simulink model "Vienna"  (R2024b)
settings: Solver=ode23t  StartTime=0.0  StopTime=2  RelTol=1e-3
undefined symbols (not defined in the file): acdc, Cur_loop_upper_limit_acdc, DiscIntNeverNeededParam, kp_ff, kr_ff, Tsim, vdc_fbk_filter
libraries: simulink x9, spsDiodeLib x6, spsMosfetLib x6, spsSeriesRLCBranchLib x5, spsVoltageMeasurementLib x4, spsMeanLib x4, spsCurrentMeasurementLib x3, spsControlledVoltageSourceLib x3, spsRMSLib x2, spsThreePhaseSourceLib x1, spsTHDLib x1, spsTriangleGeneratorLib x1
(part 1 of 2)
settings Model: Creator=PAGHDMD  LastModifiedBy=PAGHDMD
settings OptimizationCC: ReuseModelBlockBuffer=off
settings RTWCC: GPUComputeCapability=3.5

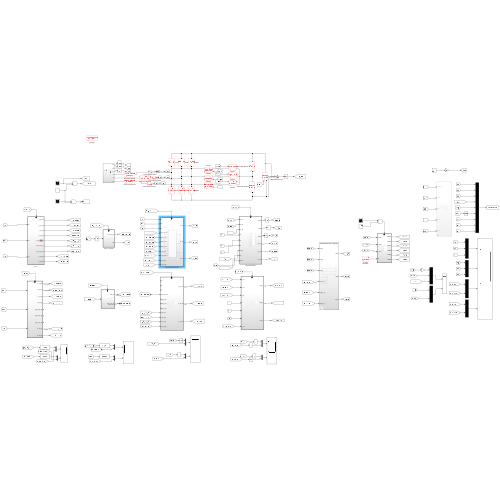
[thumbnail: Simulink's stored preview of the top-level diagram]
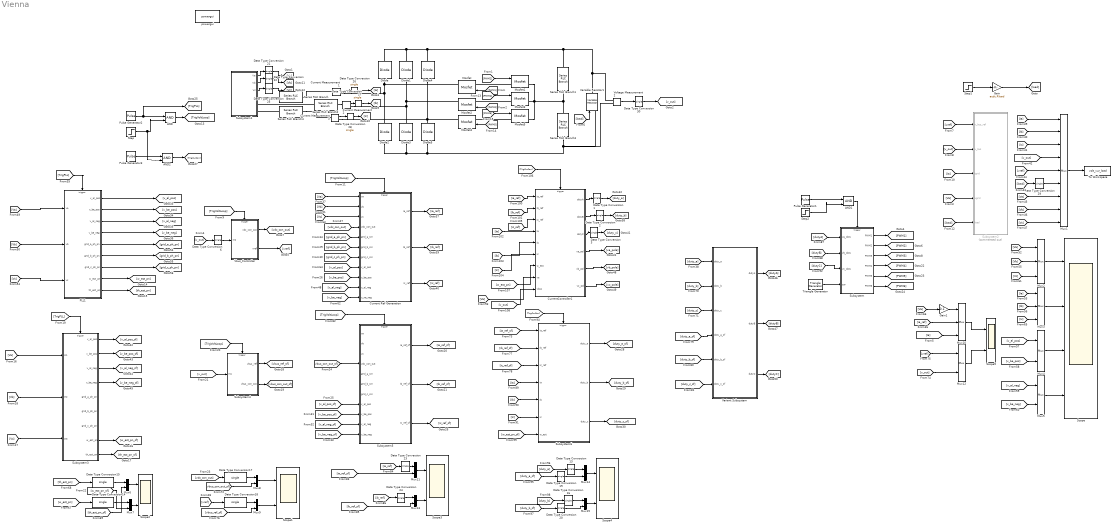
== system Vienna ==
  AND : Logic  IconShape=distinctive  AllPortsSameDT=off  OutDataTypeStr=boolean
  AND1 : Logic  IconShape=distinctive  AllPortsSameDT=off  OutDataTypeStr=boolean
  AND2 : Logic  IconShape=distinctive  AllPortsSameDT=off  OutDataTypeStr=boolean
  Current Measurement1 : spsCurrentMeasurementLib/Current Measurement  PhasorSimulation=off  OutputType=Complex  PSBequivalent=0
  Current Measurement2 : spsCurrentMeasurementLib/Current Measurement  PhasorSimulation=off  OutputType=Complex  PSBequivalent=0
  Current Measurement3 : spsCurrentMeasurementLib/Current Measurement  PhasorSimulation=off  OutputType=Complex  PSBequivalent=0
  Current Ref Generation : Subsystem
  CurrentController1 : Subsystem
  Data Type Conversion{1..3,6,13..30} (22 alike) : DataTypeConversion  OutDataTypeStr=single  SaturateOnIntegerOverflow=off  RndMeth=Floor
  Diode{,1..5} (6 alike) : spsDiodeLib/Diode  Ron=0.001  Lon=0  Vf=0.8  IC=0  UseSnubber=0  Rs=500  Cs=250e-9  Measurements=off
  Gain : Gain  Gain=acdc.Rload
  Gain1 : Gain  Gain=0.1
  Mosfet{,1..5} (6 alike) : spsMosfetLib/Mosfet  Ron=50e-3  Lon=0  Rd=0.01  Vfd=0  IC=0  Rs=1e5  Cs=inf  Measurements=on
  Mux1 : Mux  Inputs=9
  Mux10 : Mux  Inputs=3
  Mux{4..9,11..15} (11 alike) : Mux  Inputs=2
  Mux2 : Mux  Inputs=3
  Mux3 : Mux  Inputs=3
  PLL1 : Subsystem
  Pulse Generator1 : DiscretePulseGenerator  PulseType=Time based  Period=Tsim  PulseWidth=5
  Pulse Generator2 : DiscretePulseGenerator  PulseType=Time based  Period=acdc.Tvolt_loop  PulseWidth=5
  Pulse Generator3 : DiscretePulseGenerator  PulseType=Time based  Period=acdc.Tcur_loop  PulseWidth=5
  Scope : Scope  NumInputPorts=4
  Scope{1..5} (5 alike) : Scope  NumInputPorts=2
  Series RLC Branch : spsSeriesRLCBranchLib/Series RLC Branch  LConnTagsString=__new0  RConnTagsString=__new0  BranchType=RL  Resistance=acdc.L_ESR  Inductance=acdc.L  SetiL0=off  InitialCurrent=0  Capacitance=1e-6  Setx0=off  InitialVoltage=0  Measurements=None
  Series RLC Branch1 : spsSeriesRLCBranchLib/Series RLC Branch  LConnTagsString=__new0  RConnTagsString=__new0  BranchType=C  Resistance=1  Inductance=40e-6  SetiL0=off  InitialCurrent=0  Capacitance=acdc.C/2  Setx0=on  InitialVoltage=acdc.Vac_ll_rms*sqrt(2)/2  Measurements=None
  Series RLC Branch2 : spsSeriesRLCBranchLib/Series RLC Branch  LConnTagsString=__new0  RConnTagsString=__new0  BranchType=RL  Resistance=acdc.L_ESR  Inductance=acdc.L  SetiL0=off  InitialCurrent=0  Capacitance=1e-6  Setx0=off  InitialVoltage=0  Measurements=None
  Series RLC Branch3 : spsSeriesRLCBranchLib/Series RLC Branch  LConnTagsString=__new0  RConnTagsString=__new0  BranchType=C  Resistance=1  Inductance=40e-6  SetiL0=off  InitialCurrent=0  Capacitance=acdc.C/2  Setx0=on  InitialVoltage=acdc.Vac_ll_rms*sqrt(2)/2  Measurements=None
  Series RLC Branch4 : spsSeriesRLCBranchLib/Series RLC Branch  LConnTagsString=__new0  RConnTagsString=__new0  BranchType=RL  Resistance=acdc.L_ESR  Inductance=acdc.L  SetiL0=off  InitialCurrent=0  Capacitance=1e-6  Setx0=off  InitialVoltage=0  Measurements=None
  Step : Step  Time=0.02  SampleTime=0
  Step1 : Step  Time=0.5  Before=1  After=2  SampleTime=0
  Step2 : Step  Time=0.02  SampleTime=0
  Subsystem : Subsystem
  Subsystem1 : Subsystem
  Subsystem2 : Subsystem  Commented=on
  Subsystem3 : Subsystem
  Subsystem4 : Subsystem
  Subsystem5 : Subsystem
  Subsystem6 : Subsystem
  To Workspace : ToWorkspace  VariableName=volt_vur_load  SaveFormat=Timeseries  SampleTime=-1
      settings: Decimation=100
  Triangle Generator : spsTriangleGeneratorLib/Triangle Generator  Freq=acdc.Fs  Phase=0  Ts=Tsim
  Variable Resistor1 : spsVariableResistorLib/Variable Resistor  Rabsmin=1e-3
      settings: LibrarySourceBlock=sps_lib/Passives/Variable Resistor
  Variant Subsystem : Subsystem  Variant=on
  Vbus_Controller : Subsystem
  Voltage Measurement2 : spsVoltageMeasurementLib/Voltage Measurement  PhasorSimulation=off  OutputType=Complex  PSBequivalent=0
  powergui : spspowerguiLib/powergui  Priority=1  SimulationMode=Discrete  SampleTime=Tsim  frequency=60  Iterations=50  frequencyindice=0  Pbase=100e6  ErrMax=1e-4  UnitsV=kV  UnitsW=MW  buscounter=0  FunctionMessages=off  echomessages=off  EnableUseOfTLC=off  CurrentSourceSwitches=off  DisableSnubberDevices=off  DisableRonSwitches=off  DisableVfSwitches=off  DisplayEquations=off  AutomaticDiscreteSolvers=off  SolverType=Tustin/Backward Euler (TBE)  Interpol=off  ExternalGateDelay=off  methode=off  Ts=100  x0status=blocks  SPID=on  SwTol=0  HookPort=off  NonlinearTolerance=1e-4  nMaxIteration=100  ContinueOnMaxIteration=off  RestoreLinks=warning  ResistiveCurrentMeasurement=off  Frange=[0:2:500]  Ylog=off  Xlog=on  ShowGrid=off  save=off  variable=ZData  structure=0  ZoomFFT=off  StartTime=0.0  cycles=1  DisplayStyle=1  fundamental=60  FreqAxis=off  MaxFrequency=1000  frequencyindicesteady=1  RmsSteady=1  display=off
  wires:
  Voltage Measurement2/1 -> Data Type Conversion30/1
  Current Measurement1/1 -> Data Type Conversion26/1
  [PWM1] -> Mosfet/1
  [PWM2] -> Mosfet1/1
  Subsystem/1(PWM1) -> [PWM1]
  Subsystem/2(PWM2) -> [PWM2]
  Step1/1 -> Gain/1
  Gain/1 -> [load]
  [load] -> Variable Resistor1/1
  [vref] -> Subsystem2/1(v_bus_ref)
  [v_out] -> Subsystem2/2(v_bus)
  [Ia] -> Subsystem2/3(igrid)
  [Va] -> Subsystem2/4(vgrid)
  [load] -> Subsystem2/5(load)
  [v_out] -> Data Type Conversion6/1
  Vbus_Controller/2(vref) -> [vref]
  Subsystem1/1(Va) -> Data Type Conversion21/1
  [PWM3] -> Mosfet2/1
  [PWM4] -> Mosfet3/1
  [PWM5] -> Mosfet4/1
  [PWM6] -> Mosfet5/1
  Current Measurement2/1 -> Data Type Conversion27/1
  Current Measurement3/1 -> Data Type Conversion28/1
  Subsystem1/2(Vb) -> Data Type Conversion22/1
  Subsystem1/3(Vc) -> Data Type Conversion25/1
  Pulse Generator2/1 -> [TrigPLL], AND/1
  AND/1 -> [TrigVoltLoop]
  [TrigVoltLoop] -> Vbus_Controller/Trigger
  Subsystem/3(PWM3) -> [PWM3]
  Subsystem/4(PWM4) -> [PWM4]
  Subsystem/5(PWM5) -> [PWM5]
  Subsystem/6(PWM6) -> [PWM6]
  Pulse Generator1/1 -> AND1/1
  Triangle Generator/1 -> Subsystem/4(car)
  [Ia] -> Mux1/1
  [Ib] -> Mux1/2
  [Ic] -> Mux1/3
  [v_out] -> Mux1/4
  [load] -> Data Type Conversion29/1
  Mux1/1 -> To Workspace/1
  [vref] -> Mux1/5
  [Va] -> Mux1/7
  [Vb] -> Mux1/8
  [Vc] -> Mux1/9
  [TrigPLL] -> PLL1/Trigger
  Mux2/1 -> Scope/1
  [Va] -> Mux2/1
  [Vb] -> Mux2/2
  [v_al_pos] -> Mux4/1
  [v_be_pos] -> Mux4/2
  [v_al_neg] -> Mux5/1
  [v_be_neg] -> Mux5/2
  Mux3/1 -> Scope/2
  Mux4/1 -> Scope/3
  Mux5/1 -> Scope/4
  [Vc] -> Mux2/3
  [dutyA] -> Subsystem/1(va_duty)
  [dutyB] -> Subsystem/2(vb_duty)
  [dutyC] -> Subsystem/3(vc_duty)
  Mux10/1 -> Scope5/1
  [ia_ref] -> Mux10/2
  [Va] -> Gain1/1
  Gain1/1 -> Mux10/1
  Vbus_Controller/1(vdc_con_out) -> [vdc_con_out]
  [Ia] -> Mux10/3
  [TrigVoltLoop] -> Current Ref Generation/Trigger
  Current Ref Generation/1(ia_ref) -> [ia_ref]
  Current Ref Generation/2(ib_ref) -> [ib_ref]
  Current Ref Generation/3(ic_ref) -> [ic_ref]
  [vdc_con_out] -> Current Ref Generation/4(vdc_con_out)
  [grid_a_ph_pn] -> Current Ref Generation/5(grid_a_sin)
  [grid_b_ph_pn] -> Current Ref Generation/6(grid_b_sin)
  [grid_c_ph_pn] -> Current Ref Generation/7(grid_c_sin)
  Mux12/1 -> Scope5/2
  [v_out] -> Mux12/2
  [vref] -> Mux12/1
  Step2/1 -> AND1/2
  AND1/1 -> Subsystem/Trigger
  [v_al_pos] -> Current Ref Generation/8(v_al_pos)
  [v_be_pos] -> Current Ref Generation/9(v_be_pos)
  [v_al_neg] -> Current Ref Generation/10(v_al_neg)
  [v_be_neg] -> Current Ref Generation/11(v_ne_neg)
  [Ia] -> Mux3/1
  [Ib] -> Mux3/2
  [Ic] -> Mux3/3
  [Va] -> PLL1/1(va)
  [Vb] -> PLL1/2(vb)
  [Vc] -> PLL1/3(vc)
  PLL1/1(v_al_pos) -> [v_al_pos]
  PLL1/2(v_be_pos) -> [v_be_pos]
  PLL1/3(v_al_neg) -> [v_al_neg]
  PLL1/5(grid_a_ph_pn) -> [grid_a_ph_pn]
  PLL1/4(v_be_neg) -> [v_be_neg]
  PLL1/6(grid_b_ph_pn) -> [grid_b_ph_pn]
  PLL1/7(grid_c_ph_pn) -> [grid_c_ph_pn]
  [Va] -> Subsystem3/1(In1)
  [Vb] -> Subsystem3/2(In2)
  [Vc] -> Subsystem3/3(In3)
  [TrigPLL] -> Subsystem3/Trigger
  PLL1/8(w_est_pn) -> [w_est_pn]
  PLL1/9(th_est_pn) -> [th_est_pn]
  Mux7/1 -> Scope2/2
  Mux6/1 -> Scope2/1
  Data Type Conversion14/1 -> Mux7/1
  Data Type Conversion15/1 -> Mux6/1
  [TrigVoltLoop] -> Subsystem4/Trigger
  [vdc_con_out] -> Data Type Conversion17/1
  Mux8/1 -> Scope1/1
  [v_out] -> Subsystem4/1(In1)
  Data Type Conversion17/1 -> Mux8/1
  Mux9/1 -> Scope1/2
  [vref] -> Data Type Conversion18/1
  Data Type Conversion18/1 -> Mux9/1
  [w_est_pn] -> Data Type Conversion14/1
  [th_est_pn] -> Data Type Conversion15/1
  Subsystem3/8(w_est_pn) -> [w_est_pn_sf]
  Subsystem3/9(th_est_pn) -> [th_est_pn_sf]
  [w_est_pn_sf] -> Mux7/2
  [th_est_pn_sf] -> Mux6/2
  Subsystem4/2(vbus_con_out) -> [vbus_con_out_sf]
  Subsystem4/1(vbus_ref) -> [vbus_ref_sf]
  [vbus_con_out_sf] -> Mux8/2
  [vbus_ref_sf] -> Mux9/2
  Subsystem5/1(ia_ref_sf) -> [ia_ref_sf]
  Subsystem5/2(ib_ref_sf) -> [ib_ref_sf]
  Subsystem5/3(ic_ref_sf) -> [ic_ref_sf]
  [TrigVoltLoop] -> Subsystem5/Trigger
  [v_al_pos_sf] -> Subsystem5/8(v_al_pos)
  [v_be_pos_sf] -> Subsystem5/9(v_be_pos)
  [v_al_neg_sf] -> Subsystem5/10(v_al_neg)
  [v_be_neg_sf] -> Subsystem5/11(v_be_neg)
  Mux11/1 -> Scope3/1
  Mux13/1 -> Scope3/2
  [ia_ref] -> Data Type Conversion23/1
  [ia_ref_sf] -> Mux11/2
  [ib_ref_sf] -> Mux13/2
  [vbus_con_out_sf] -> Subsystem5/4(vdc_con_out)
  Data Type Conversion23/1 -> Mux11/1
  [ib_ref] -> Data Type Conversion24/1
  Data Type Conversion24/1 -> Mux13/1
  [ib_ref_sf] -> Subsystem6/2(ib_ref)
  [ic_ref_sf] -> Subsystem6/3(ic_ref)
  [ia_ref_sf] -> Subsystem6/1(ia_ref)
  [Ia] -> Subsystem6/4(ia)
  [Ib] -> Subsystem6/5(ib)
  [Ic] -> Subsystem6/6(ic)
  Pulse Generator3/1 -> AND2/1
  Step/1 -> AND2/2, AND/2
  AND2/1 -> [TrigCurCon]
  [TrigCurCon] -> Subsystem6/Trigger
  Subsystem6/1(duty_a) -> [duty_a_sf]
  Subsystem6/2(duty_b) -> [duty_b_sf]
  Subsystem6/3(duty_c) -> [duty_c_sf]
  [duty_a_sf] -> Data Type Conversion19/1
  [duty_b_sf] -> Data Type Conversion20/1
  Mux15/1 -> Scope4/2
  Mux14/1 -> Scope4/1
  [duty_b] -> Data Type Conversion16/1
  [duty_a] -> Data Type Conversion13/1
  [w_est_pn_sf] -> Subsystem6/7(w_est)
  CurrentController1/4(va_pol) -> [va_pole]
  CurrentController1/3(dutyC) -> Data Type Conversion3/1
  [w_est_pn] -> CurrentController1/7(w_est)
  CurrentController1/6(vc_pol) -> [vc_pole]
  CurrentController1/1(dutyA) -> Data Type Conversion1/1
  [ib_ref] -> CurrentController1/2(ib_ref)
  [ic_ref] -> CurrentController1/3(ic_ref)
  CurrentController1/5(vb_pol) -> [vb_pole]
  [ia_ref] -> CurrentController1/1(ia_ref)
  CurrentController1/2(dutyB) -> Data Type Conversion2/1
  [TrigCurCon] -> CurrentController1/Trigger
  Subsystem3/1(v_al_pos) -> [v_al_pos_sf]
  Subsystem3/2(v_be_pos) -> [v_be_pos_sf]
  Subsystem3/3(v_al_neg) -> [v_al_neg_sf]
  Subsystem3/4(v_be_neg) -> [v_be_neg_sf]
  Data Type Conversion13/1 -> Mux14/1
  Data Type Conversion16/1 -> Mux15/1
  Data Type Conversion19/1 -> Mux14/2
  Data Type Conversion20/1 -> Mux15/2
  [Va] -> Current Ref Generation/1(va)
  [Vb] -> Current Ref Generation/2(vb)
  [Vc] -> Current Ref Generation/3(vc)
  Data Type Conversion6/1 -> Vbus_Controller/1(In2)
  [Ia] -> CurrentController1/4(ia)
  [Ib] -> CurrentController1/5(ib)
  [Ic] -> CurrentController1/6(ic)
  Data Type Conversion21/1 -> [Va]
  Data Type Conversion22/1 -> [Vb]
  Data Type Conversion25/1 -> [Vc]
  Data Type Conversion26/1 -> [Ia]
  Data Type Conversion27/1 -> [Ib]
  Data Type Conversion28/1 -> [Ic]
  Data Type Conversion29/1 -> Mux1/6
  Data Type Conversion30/1 -> [v_out]
  Data Type Conversion1/1 -> [duty_a]
  Data Type Conversion2/1 -> [duty_b]
  Data Type Conversion3/1 -> [duty_c]
  [duty_c_sf] -> Variant Subsystem/6(duty_c_sf)
  [duty_a] -> Variant Subsystem/1(duty_a)
  [duty_b] -> Variant Subsystem/2(duty_b)
  [duty_c] -> Variant Subsystem/3(duty_c)
  [duty_b_sf] -> Variant Subsystem/5(duty_b_sf)
  [duty_a_sf] -> Variant Subsystem/4(duty_a_sf)
  Variant Subsystem/1(dutyA) -> [dutyA]
  Variant Subsystem/2(dutyB) -> [dutyB]
  Variant Subsystem/3(dutyC) -> [dutyC]
  [Va] -> CurrentController1/8(va)
  [v_out] -> CurrentController1/9(vbus)
  connections:
  Diode2/RConn1 -- Current Measurement1/RConn1 -- Mosfet/RConn1 -- Diode/LConn1
  Diode2/LConn1 -- Diode3/LConn1 -- Diode5/LConn1 -- Series RLC Branch3/RConn1 -- Voltage Measurement2/LConn2 -- Variable Resistor1/LConn1
  Voltage Measurement2/LConn1 -- Diode4/RConn1 -- Diode1/RConn1 -- Diode/RConn1 -- Series RLC Branch1/LConn1 -- Variable Resistor1/RConn1
  Mosfet1/RConn1 -- Series RLC Branch3/LConn1 -- Series RLC Branch1/RConn1 -- Mosfet5/RConn1 -- Mosfet3/RConn1
  Current Measurement1/LConn1 -- Series RLC Branch/RConn1
  Mosfet1/LConn1 -- Mosfet/LConn1
  Subsystem1/RConn1 -- Series RLC Branch/LConn1
  Series RLC Branch2/LConn1 -- Subsystem1/RConn2
  Series RLC Branch4/LConn1 -- Subsystem1/RConn3
  Diode1/LConn1 -- Diode3/RConn1 -- Current Measurement2/RConn1 -- Mosfet2/RConn1
  Diode4/LConn1 -- Mosfet4/RConn1 -- Current Measurement3/RConn1 -- Diode5/RConn1
  Mosfet3/LConn1 -- Mosfet2/LConn1
  Mosfet5/LConn1 -- Mosfet4/LConn1
  Series RLC Branch2/RConn1 -- Current Measurement2/LConn1
  Series RLC Branch4/RConn1 -- Current Measurement3/LConn1

== system Vienna/Current Ref Generation ==
  va : Inport
  vb : Inport  Port=2
  vc : Inport  Port=3
  vdc_con_out : Inport  Port=4
  grid_a_sin : Inport  Port=5
  grid_b_sin : Inport  Port=6
  grid_c_sin : Inport  Port=7
  v_al_pos : Inport  Port=8
  v_be_pos : Inport  Port=9
  v_al_neg : Inport  Port=10
  v_ne_neg : Inport  Port=11
  Trigger : TriggerPort  VariantControl=(inherit)  PortDimensions=1
  Variant Subsystem : Subsystem  Variant=on
  ia_ref : Outport  OutDataTypeStr=single
  ib_ref : Outport  Port=2  OutDataTypeStr=single
  ic_ref : Outport  Port=3  OutDataTypeStr=single
  wires:
  Variant Subsystem/2(ib_ref) -> ib_ref/1
  va/1 -> Variant Subsystem/1(va)
  vb/1 -> Variant Subsystem/2(vb)
  vc/1 -> Variant Subsystem/3(vc)
  vdc_con_out/1 -> Variant Subsystem/4(vdc_con_out)
  grid_a_sin/1 -> Variant Subsystem/5(grid_a_sin)
  grid_b_sin/1 -> Variant Subsystem/6(grid_b_sin)
  grid_c_sin/1 -> Variant Subsystem/7(grid_c_sin)
  Variant Subsystem/1(ia_ref) -> ia_ref/1
  Variant Subsystem/3(ic_ref) -> ic_ref/1
  v_al_pos/1 -> Variant Subsystem/8(v_al_pos)
  v_be_pos/1 -> Variant Subsystem/9(v_be_pos)
  v_al_neg/1 -> Variant Subsystem/10(v_al_neg)
  v_ne_neg/1 -> Variant Subsystem/11(v_be_neg)

== system Vienna/CurrentController1 ==
  ia_ref : Inport
  ib_ref : Inport  Port=2
  ic_ref : Inport  Port=3
  ia : Inport  Port=4
  ib : Inport  Port=5
  ic : Inport  Port=6
  w_est : Inport  Port=7
  va : Inport  Port=8
  vbus : Inport  Port=9
  Trigger : TriggerPort  VariantControl=(inherit)  PortDimensions=1
  Variant Subsystem : Subsystem  Variant=on
  dutyA : Outport
  dutyB : Outport  Port=2
  dutyC : Outport  Port=3
  va_pol : Outport  Port=4
  vb_pol : Outport  Port=5
  vc_pol : Outport  Port=6
  wires:
  ia_ref/1 -> Variant Subsystem/1(ia_ref)
  ib_ref/1 -> Variant Subsystem/2(ib_ref)
  ic_ref/1 -> Variant Subsystem/3(ic_ref)
  ib/1 -> Variant Subsystem/5(ib)
  w_est/1 -> Variant Subsystem/7(w_est)
  ia/1 -> Variant Subsystem/4(ia)
  ic/1 -> Variant Subsystem/6(ic)
  Variant Subsystem/1(dutyA) -> dutyA/1
  Variant Subsystem/2(dutyB) -> dutyB/1
  Variant Subsystem/3(dutyC) -> dutyC/1
  Variant Subsystem/4(va_pol) -> va_pol/1
  Variant Subsystem/5(vb_pol) -> vb_pol/1
  Variant Subsystem/6(vc_pol) -> vc_pol/1
  va/1 -> Variant Subsystem/8(va)
  vbus/1 -> Variant Subsystem/9(vbus)

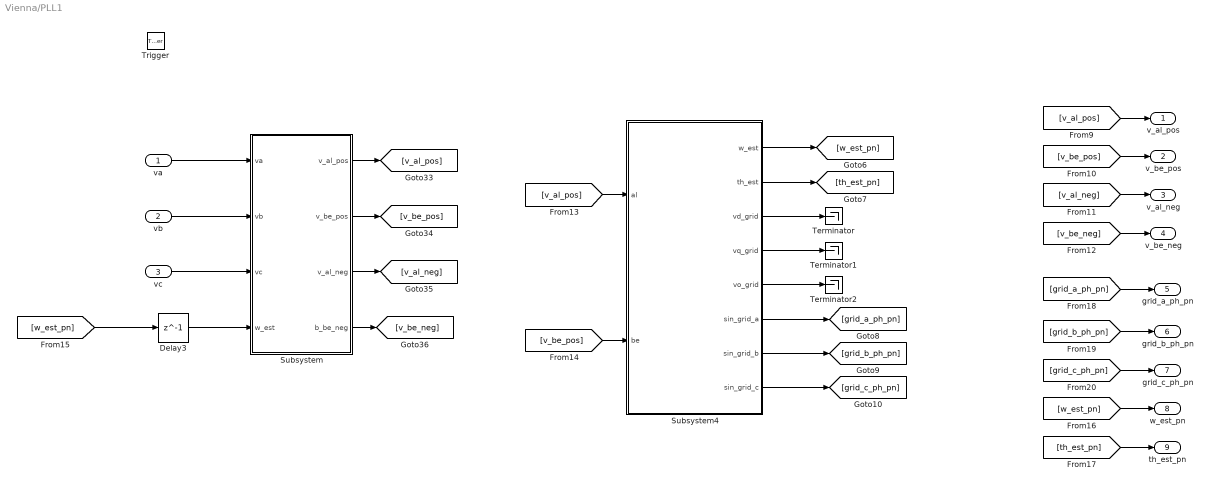
== system Vienna/PLL1 ==
  va : Inport
  vb : Inport  Port=2
  vc : Inport  Port=3
  Trigger : TriggerPort  VariantControl=(inherit)  PortDimensions=1
  Delay3 : Delay  DelayLength=1
  Subsystem : Subsystem
  Subsystem4 : Subsystem
  Terminator : Terminator
  Terminator1 : Terminator
  Terminator2 : Terminator
  v_al_pos : Outport
  v_be_pos : Outport  Port=2
  v_al_neg : Outport  Port=3
  v_be_neg : Outport  Port=4
  grid_a_ph_pn : Outport  Port=5
  grid_b_ph_pn : Outport  Port=6
  grid_c_ph_pn : Outport  Port=7
  w_est_pn : Outport  Port=8
  th_est_pn : Outport  Port=9
  wires:
  [w_est_pn] -> Delay3/1
  va/1 -> Subsystem/1(va)
  vb/1 -> Subsystem/2(vb)
  vc/1 -> Subsystem/3(vc)
  Subsystem/1(v_al_pos) -> [v_al_pos]
  Subsystem/2(v_be_pos) -> [v_be_pos]
  Subsystem/3(v_al_neg) -> [v_al_neg]
  Subsystem/4(b_be_neg) -> [v_be_neg]
  Delay3/1 -> Subsystem/4(w_est)
  [v_al_pos] -> v_al_pos/1
  [v_be_pos] -> v_be_pos/1
  [v_al_neg] -> v_al_neg/1
  [v_be_neg] -> v_be_neg/1
  [v_al_pos] -> Subsystem4/1(al)
  [v_be_pos] -> Subsystem4/2(be)
  Subsystem4/1(w_est) -> [w_est_pn]
  Subsystem4/6(sin_grid_a) -> [grid_a_ph_pn]
  Subsystem4/7(sin_grid_b) -> [grid_b_ph_pn]
  Subsystem4/8(sin_grid_c) -> [grid_c_ph_pn]
  Subsystem4/2(th_est) -> [th_est_pn]
  [w_est_pn] -> w_est_pn/1
  [th_est_pn] -> th_est_pn/1
  [grid_a_ph_pn] -> grid_a_ph_pn/1
  [grid_b_ph_pn] -> grid_b_ph_pn/1
  [grid_c_ph_pn] -> grid_c_ph_pn/1
  Subsystem4/3(vd_grid) -> Terminator/1
  Subsystem4/4(vq_grid) -> Terminator1/1
  Subsystem4/5(vo_grid) -> Terminator2/1

== system Vienna/Subsystem ==
  va_duty : Inport
  vb_duty : Inport  Port=2
  vc_duty : Inport  Port=3
  car : Inport  Port=4
  Trigger : TriggerPort  VariantControl=(inherit)  PortDimensions=1
  Variant Subsystem : Subsystem  Variant=on
  PWM1 : Outport
  PWM2 : Outport  Port=2
  PWM3 : Outport  Port=3
  PWM4 : Outport  Port=4
  PWM5 : Outport  Port=5
  PWM6 : Outport  Port=6
  wires:
  va_duty/1 -> Variant Subsystem/1(va_duty)
  vb_duty/1 -> Variant Subsystem/2(vb_duty)
  vc_duty/1 -> Variant Subsystem/3(vc_duty)
  car/1 -> Variant Subsystem/4(car)
  Variant Subsystem/1(PWM1) -> PWM1/1
  Variant Subsystem/2(PWM2) -> PWM2/1
  Variant Subsystem/3(PWM3) -> PWM3/1
  Variant Subsystem/4(PWM4) -> PWM4/1
  Variant Subsystem/5(PWM5) -> PWM5/1
  Variant Subsystem/6(PWM6) -> PWM6/1

== system Vienna/Subsystem1 ==
  Scope : Scope  NumInputPorts=3
  Subsystem : Subsystem
  Subsystem1 : Subsystem
  Three-Phase Source : spsThreePhaseSourceLib/Three-Phase Source  InternalConnection=Yn  VoltagePhases=on  Voltage=acdc.Vac_ll_rms  PhaseAngle=0  Voltage_phases="[acdc.va  acdc.vb acdc.vc]"  PhaseAngles_phases="[acdc.va_ph  acdc.vb_ph  acdc.vc_ph]"  Frequency=acdc.Fac  NonIdealSource=off  SpecifyImpedance=off  Resistance=0.8929  Inductance=16.58e-3  ShortCircuitLevel=100e6  BaseVoltage=25e3  XRratio=7  BusType=swing  Pref=10e3  Qref=0  Prefabc=[10e3, 10e3, 10e3]  Qrefabc=[0, 0, 0]  Qmin=-inf  Qmax=inf
  Voltage Measurement1 : spsVoltageMeasurementLib/Voltage Measurement  PhasorSimulation=off  OutputType=Complex  PSBequivalent=0
  Voltage Measurement2 : spsVoltageMeasurementLib/Voltage Measurement  PhasorSimulation=off  OutputType=Complex  PSBequivalent=0
  Voltage Measurement3 : spsVoltageMeasurementLib/Voltage Measurement  PhasorSimulation=off  OutputType=Complex  PSBequivalent=0
  A : PMIOPort  Side=Right
  B : PMIOPort  Port=2  Side=Right
  C : PMIOPort  Port=3  Side=Right
  Va : Outport
  Vb : Outport  Port=2
  Vc : Outport  Port=3
  wires:
  Voltage Measurement1/1 -> Va/1
  Voltage Measurement2/1 -> Vb/1
  Voltage Measurement3/1 -> Vc/1
  Subsystem1/1(s) -> Subsystem/1(s), Scope/1
  Subsystem1/2(s1) -> Subsystem/2(s1), Scope/2
  Subsystem1/3(s2) -> Subsystem/3(s2), Scope/3
  connections:
  A/RConn1 -- Subsystem/RConn1 -- Voltage Measurement1/LConn1
  Voltage Measurement3/LConn1 -- C/RConn1 -- Subsystem/RConn3
  Voltage Measurement2/LConn1 -- Subsystem/RConn2 -- B/RConn1
  Voltage Measurement1/LConn2 -- Voltage Measurement3/LConn2 -- Subsystem/RConn4 -- Voltage Measurement2/LConn2

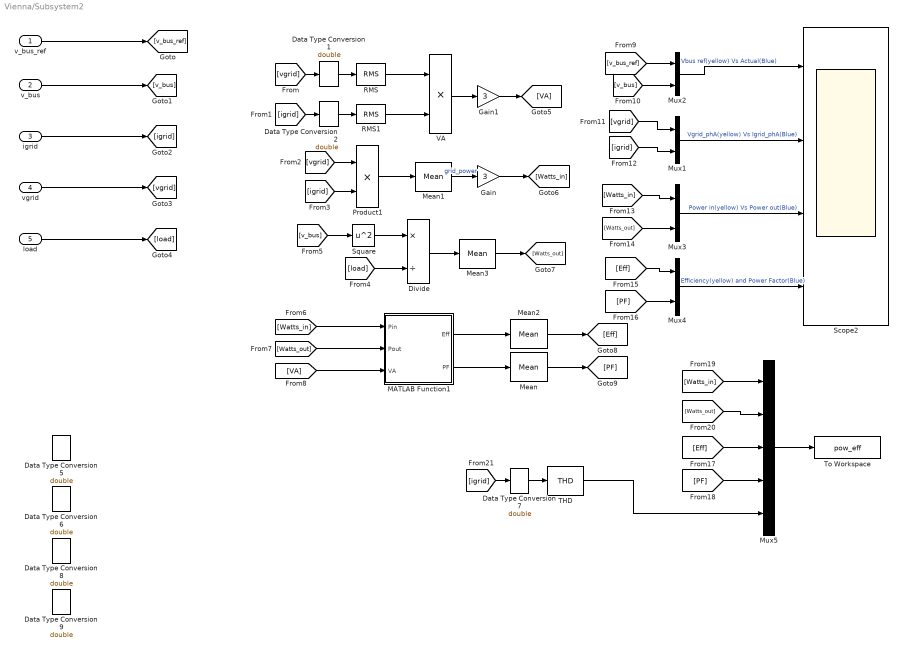
== system Vienna/Subsystem2 ==
  v_bus_ref : Inport
  v_bus : Inport  Port=2
  igrid : Inport  Port=3
  vgrid : Inport  Port=4
  load : Inport  Port=5
  Data Type Conversion{1..2,5..9} (7 alike) : DataTypeConversion  OutDataTypeStr=double  SaturateOnIntegerOverflow=off  RndMeth=Floor
  Divide : Product  Inputs=*/
  Gain : Gain  Gain=3
  Gain1 : Gain  Gain=3
  MATLAB Function1 : MATLAB Function  TreatAsAtomicUnit=on
  Mean : spsMeanLib/Mean  Freq=acdc.Fac  Vinit=0  Ts=Tsim
  Mean1 : spsMeanLib/Mean  Freq=acdc.Fac  Vinit=0  Ts=0
  Mean2 : spsMeanLib/Mean  Freq=acdc.Fac  Vinit=0  Ts=Tsim
  Mean3 : spsMeanLib/Mean  Freq=acdc.Fac  Vinit=0  Ts=Tsim
  Mux{1..4} (4 alike) : Mux  Inputs=2
  Mux5 : Mux  Inputs=5
  Product1 : Product  OutDataTypeStr=double
  RMS : spsRMSLib/RMS  TrueRMS=on  Freq=acdc.Fac  RMSInit=0  Ts=0
  RMS1 : spsRMSLib/RMS  TrueRMS=on  Freq=acdc.Fac  RMSInit=0  Ts=0
  Scope2 : Scope  NumInputPorts=4
  Square : Math  Operator=square
  THD : spsTHDLib/THD  Freq=60  Ts=Tsim
  To Workspace : ToWorkspace  VariableName=pow_eff  SaveFormat=Timeseries  SampleTime=-1
      settings: Decimation=100
  VA : Product  OutDataTypeStr=single
  wires:
  Square/1 -> Divide/1
  Divide/1 -> Mean3/1
  Mux1/1 -> Scope2/2  "Vgrid_phA(yellow) Vs Igrid_phA(Blue)"
  Product1/1 -> Mean1/1
  Mux2/1 -> Scope2/1  "Vbus ref(yellow) Vs Actual(Blue)"
  Mean1/1 -> Gain/1  "grid_power"
  Gain/1 -> [Watts_in]
  RMS/1 -> VA/1
  RMS1/1 -> VA/2
  VA/1 -> Gain1/1
  Gain1/1 -> [VA]
  [vgrid] -> Data Type Conversion1/1
  [igrid] -> Data Type Conversion2/1
  [vgrid] -> Product1/1
  [igrid] -> Product1/2
  [load] -> Divide/2
  [v_bus] -> Square/1
  Mux3/1 -> Scope2/3  "Power in(yellow) Vs Power out(Blue)"
  [Watts_in] -> MATLAB Function1/1(Pin)
  [Watts_out] -> MATLAB Function1/2(Pout)
  MATLAB Function1/1(Eff) -> Mean2/1
  [VA] -> MATLAB Function1/3(VA)
  MATLAB Function1/2(PF) -> Mean/1
  Mux4/1 -> Scope2/4  "Efficiency(yellow) and Power Factor(Blue)"
  [v_bus_ref] -> Mux2/1
  [v_bus] -> Mux2/2
  [vgrid] -> Mux1/1
  [igrid] -> Mux1/2
  [Watts_in] -> Mux3/1
  [Watts_out] -> Mux3/2
  [Eff] -> Mux4/1
  [PF] -> Mux4/2
  Mean/1 -> [PF]
  Mean2/1 -> [Eff]
  Mean3/1 -> [Watts_out]
  Mux5/1 -> To Workspace/1
  [Watts_in] -> Mux5/1
  [Watts_out] -> Mux5/2
  [Eff] -> Mux5/3
  [PF] -> Mux5/4
  [igrid] -> Data Type Conversion7/1
  THD/1 -> Mux5/5
  v_bus_ref/1 -> [v_bus_ref]
  v_bus/1 -> [v_bus]
  igrid/1 -> [igrid]
  vgrid/1 -> [vgrid]
  load/1 -> [load]
  Data Type Conversion1/1 -> RMS/1
  Data Type Conversion2/1 -> RMS1/1
  Data Type Conversion7/1 -> THD/1

== system Vienna/Subsystem3 ==
  In1 : Inport
  In2 : Inport  Port=2
  In3 : Inport  Port=3
  Trigger : TriggerPort  VariantControl=(inherit)  PortDimensions=1
  Bus Creator : BusCreator  Inputs=3
  Bus Selector : BusSelector  OutputSignals=seq_comps.v_al_pos,seq_comps.v_be_pos,seq_comps.v_al_neg,seq_comps.v_be_neg,th_est,w_est,debug1,debug2
  S-Function : S-Function  FunctionName=sfun_pll  SFunctionDeploymentMode=off  EnableBusSupport=off
  Scope2 : Scope  NumInputPorts=3
  v_al_pos : Outport
  v_be_pos : Outport  Port=2
  v_al_neg : Outport  Port=3
  v_be_neg : Outport  Port=4
  grid_a_ph_pn : Outport  Port=5
  grid_b_ph_pn : Outport  Port=6
  grid_c_ph_pn : Outport  Port=7
  w_est_pn : Outport  Port=8
  th_est_pn : Outport  Port=9
  wires:
  In3/1 -> Bus Creator/3
  In2/1 -> Scope2/3, Bus Creator/2
  In1/1 -> Bus Creator/1
  ? -> grid_c_ph_pn/1
  ? -> grid_b_ph_pn/1
  ? -> grid_a_ph_pn/1
  Bus Selector/5 -> th_est_pn/1  "<th_est>"
  Bus Selector/6 -> w_est_pn/1  "<w_est>"
  Bus Selector/1 -> v_al_pos/1  "<v_al_pos>"
  Bus Selector/3 -> v_al_neg/1  "<v_al_neg>"
  Bus Selector/7 -> Scope2/1  "<debug1>"
  Bus Selector/8 -> Scope2/2  "<debug2>"
  Bus Creator/1 -> S-Function/1
  S-Function/1 -> Bus Selector/1
  Bus Selector/2 -> v_be_pos/1  "<v_be_pos>"
  Bus Selector/4 -> v_be_neg/1  "<v_be_neg>"

== system Vienna/Subsystem4 ==
  In1 : Inport
  Trigger : TriggerPort  VariantControl=(inherit)  PortDimensions=1
  Bus Creator : BusCreator  Inputs=1
  Bus Selector : BusSelector  OutputSignals=vbus_ref,vbus_con_out,debug1,debug2
  Data Type Conversion16 : DataTypeConversion  OutDataTypeStr=single  SaturateOnIntegerOverflow=off  RndMeth=Floor
  S-Function : S-Function  FunctionName=sfun_vbus_con  SFunctionDeploymentMode=off  EnableBusSupport=off
  Scope2 : Scope  NumInputPorts=3
  vbus_ref : Outport
  vbus_con_out : Outport  Port=2
  wires:
  In1/1 -> Data Type Conversion16/1
  Bus Selector/1 -> vbus_ref/1  "<vbus_ref>"
  Bus Selector/2 -> vbus_con_out/1  "<vbus_con_out>"
  Bus Selector/4 -> Scope2/2  "<debug2>"
  Bus Creator/1 -> S-Function/1
  S-Function/1 -> Bus Selector/1
  Bus Selector/3 -> Scope2/1  "<debug1>"
  Data Type Conversion16/1 -> Bus Creator/1

== system Vienna/Subsystem5 ==
  va : Inport
  vb : Inport  Port=2
  vc : Inport  Port=3
  vdc_con_out : Inport  Port=4
  grid_a_sin : Inport  Port=5
  grid_b_sin : Inport  Port=6
  grid_c_sin : Inport  Port=7
  v_al_pos : Inport  Port=8
  v_be_pos : Inport  Port=9
  v_al_neg : Inport  Port=10
  v_be_neg : Inport  Port=11
  Trigger : TriggerPort  VariantControl=(inherit)  PortDimensions=1
  Bus Creator : BusCreator  Inputs=4  OutDataTypeStr=Bus: CURREFGEN_IN_TYPE
  Bus Creator2 : BusCreator  Inputs=3
  Bus Creator3 : BusCreator  Inputs=3
  Bus Creator4 : BusCreator  Inputs=4
  Bus Selector : BusSelector  OutputSignals=iabc.A,iabc.B,iabc.C,debug1,debug2
  S-Function : S-Function  FunctionName=sfun_cur_ref_gen  SFunctionDeploymentMode=off  EnableBusSupport=off
  Scope2 : Scope  NumInputPorts=3
  ia_ref_sf : Outport
  ib_ref_sf : Outport  Port=2
  ic_ref_sf : Outport  Port=3
  wires:
  Bus Selector/1 -> ia_ref_sf/1  "<A>"
  Bus Selector/2 -> ib_ref_sf/1  "<B>"
  Bus Selector/5 -> Scope2/2  "<debug2>"
  Bus Creator/1 -> S-Function/1
  S-Function/1 -> Bus Selector/1
  Bus Selector/4 -> Scope2/1  "<debug1>"
  vb/1 -> Bus Creator2/2
  va/1 -> Bus Creator2/1
  vc/1 -> Bus Creator2/3
  grid_c_sin/1 -> Bus Creator3/3
  grid_b_sin/1 -> Bus Creator3/2
  grid_a_sin/1 -> Bus Creator3/1
  Bus Creator2/1 -> Bus Creator/2
  Bus Creator4/1 -> Bus Creator/3
  Bus Creator3/1 -> Bus Creator/4
  Bus Selector/3 -> ic_ref_sf/1  "<C>"
  v_al_pos/1 -> Bus Creator4/1
  v_al_neg/1 -> Bus Creator4/2
  v_be_pos/1 -> Bus Creator4/3
  v_be_neg/1 -> Bus Creator4/4
  vdc_con_out/1 -> Bus Creator/1

== system Vienna/Subsystem6 ==
  ia_ref : Inport
  ib_ref : Inport  Port=2
  ic_ref : Inport  Port=3
  ia : Inport  Port=4
  ib : Inport  Port=5
  ic : Inport  Port=6
  w_est : Inport  Port=7
  Trigger : TriggerPort  VariantControl=(inherit)  PortDimensions=1
  Bus Creator : BusCreator  Inputs=3  OutDataTypeStr=Bus: CURCONTROLLER_IN_TYPE
  Bus Creator2 : BusCreator  Inputs=3  OutDataTypeStr=Bus: ABC_TYPE
  Bus Creator3 : BusCreator  Inputs=3  OutDataTypeStr=Bus: ABC_TYPE
  Bus Selector : BusSelector  OutputSignals=duty_abc.A,duty_abc.B,duty_abc.C,debug1,debug2
  Data Type Conversion1 : DataTypeConversion  OutDataTypeStr=double  SaturateOnIntegerOverflow=off  RndMeth=Floor
  Data Type Conversion8 : DataTypeConversion  OutDataTypeStr=double  SaturateOnIntegerOverflow=off  RndMeth=Floor
  Data Type Conversion9 : DataTypeConversion  OutDataTypeStr=double  SaturateOnIntegerOverflow=off  RndMeth=Floor
  S-Function : S-Function  FunctionName=sfun_cur_con  SFunctionDeploymentMode=off  EnableBusSupport=off
  Scope2 : Scope  NumInputPorts=3
  duty_a : Outport
  duty_b : Outport  Port=2
  duty_c : Outport  Port=3
  wires:
  Bus Selector/1 -> Data Type Conversion1/1  "<A>"
  Bus Selector/2 -> Data Type Conversion8/1  "<B>"
  Bus Selector/5 -> Scope2/2  "<debug2>"
  Bus Creator/1 -> S-Function/1
  S-Function/1 -> Bus Selector/1
  Bus Selector/4 -> Scope2/1  "<debug1>"
  Bus Selector/3 -> Data Type Conversion9/1  "<C>"
  Bus Creator2/1 -> Bus Creator/1
  Bus Creator3/1 -> Bus Creator/2
  ia_ref/1 -> Bus Creator2/1
  ib_ref/1 -> Bus Creator2/2
  ic_ref/1 -> Bus Creator2/3
  ia/1 -> Bus Creator3/1
  ib/1 -> Bus Creator3/2
  ic/1 -> Bus Creator3/3
  w_est/1 -> Bus Creator/3
  Data Type Conversion1/1 -> duty_a/1
  Data Type Conversion8/1 -> duty_b/1
  Data Type Conversion9/1 -> duty_c/1

== system Vienna/Variant Subsystem ==
  duty_a : Inport
  duty_b : Inport  Port=2
  duty_c : Inport  Port=3
  duty_a_sf : Inport  Port=4
  duty_b_sf : Inport  Port=5
  duty_c_sf : Inport  Port=6
  S FUNCTION CONTROL : Subsystem  VariantControl=sfunc_based_con == 1
  SIMULINK BLOCK CONTROL : Subsystem  VariantControl=sfunc_based_con == 0
  dutyA : Outport
  dutyB : Outport  Port=2
  dutyC : Outport  Port=3

== system Vienna/Vbus_Controller ==
  In2 : Inport
  Trigger : TriggerPort  VariantControl=(inherit)  PortDimensions=1
  Add : Sum  Inputs=+-
  Constant : Constant  Value=acdc.Vac_ph_pk*sqrt(3)  OutDataTypeStr=single
  Constant1 : Constant  Value=acdc.Tvolt_loop  OutDataTypeStr=single
  Constant2 : Constant  Value=vdc_fbk_filter  OutDataTypeStr=single
  Delay3 : Delay  DelayLength=1  InitialCondition=acdc.Vac_ph_pk*sqrt(3)
  Discrete Transfer Fcn : DiscreteTransferFcn  Numerator=acdc.notch_num  Denominator=acdc.notch_den
  MATLAB Function4 : MATLAB Function  TreatAsAtomicUnit=on
  PI : Subsystem
  Saturation : Saturate  UpperLimit=acdc.vdc_con_max  LowerLimit=acdc.vdc_con_min
  Saturation2 : Saturate  UpperLimit=acdc.Vref  LowerLimit=0
  Scope1 : Scope  NumInputPorts=3
  Switch : Switch  Criteria=u2 ~= 0  Threshold=1  SaturateOnIntegerOverflow=off  InputSameDT=off
  vdc_con_out : Outport
  vref : Outport  Port=2
  wires:
  Saturation/1 -> Scope1/2, vdc_con_out/1
  Saturation2/1 -> vref/1, Add/1
  Add/1 -> Scope1/1, PI/1(q)
  PI/1(Out1) -> Saturation/1
  MATLAB Function4/1(vdc_ref) -> Saturation2/1, Delay3/1
  In2/1 -> Discrete Transfer Fcn/1, Switch/3
  Constant1/1 -> MATLAB Function4/2(Tcon)
  Constant/1 -> MATLAB Function4/1(vdc_max)
  Delay3/1 -> MATLAB Function4/3(vdc_old)
  Switch/1 -> Add/2
  Discrete Transfer Fcn/1 -> Switch/1
  Constant2/1 -> Switch/2

== system Vienna/Current Ref Generation/Variant Subsystem ==
  va : Inport
  vb : Inport  Port=2
  vc : Inport  Port=3
  vdc_con_out : Inport  Port=4
  grid_a_sin : Inport  Port=5
  grid_b_sin : Inport  Port=6
  grid_c_sin : Inport  Port=7
  v_al_pos : Inport  Port=8
  v_be_pos : Inport  Port=9
  v_al_neg : Inport  Port=10
  v_be_neg : Inport  Port=11
  current control : Subsystem  VariantControl=power_base_control == 0
  power control : Subsystem  VariantControl=power_base_control == 1
  power control seq comp : Subsystem  VariantControl=power_base_control == 2
  ia_ref : Outport
  ib_ref : Outport  Port=2
  ic_ref : Outport  Port=3

== system Vienna/CurrentController1/Variant Subsystem ==
  ia_ref : Inport
  ib_ref : Inport  Port=2
  ic_ref : Inport  Port=3
  ia : Inport  Port=4
  ib : Inport  Port=5
  ic : Inport  Port=6
  w_est : Inport  Port=7
  va : Inport  Port=8
  vbus : Inport  Port=9
  PR : Subsystem  VariantControl=sogi_pr == 0
  SOGI_PR : Subsystem  VariantControl=sogi_pr == 1
  SOGI_PR_FF : Subsystem  VariantControl=sogi_pr == 2
  dutyA : Outport
  dutyB : Outport  Port=2
  dutyC : Outport  Port=3
  va_pol : Outport  Port=4
  vb_pol : Outport  Port=5
  vc_pol : Outport  Port=6

== system Vienna/PLL1/Subsystem ==
  va : Inport
  vb : Inport  Port=2
  vc : Inport  Port=3
  w_est : Inport  Port=4
  Data Type Conversion : DataTypeConversion  OutDataTypeStr=single  SaturateOnIntegerOverflow=off  RndMeth=Floor
  Data Type Conversion1 : DataTypeConversion  OutDataTypeStr=single  SaturateOnIntegerOverflow=off  RndMeth=Floor
  Data Type Conversion2 : DataTypeConversion  OutDataTypeStr=single  SaturateOnIntegerOverflow=off  RndMeth=Floor
  SOGI : Subsystem
  Sequence Comps : Subsystem
  v_al_pos : Outport
  v_be_pos : Outport  Port=2
  v_al_neg : Outport  Port=3
  b_be_neg : Outport  Port=4
  wires:
  Sequence Comps/2(v_be_pos) -> v_be_pos/1
  Sequence Comps/4(v_be_neg) -> b_be_neg/1
  SOGI/1(al) -> Sequence Comps/1(v_al)
  SOGI/3(be) -> Sequence Comps/3(v_be)
  SOGI/2(q_al) -> Sequence Comps/2(qv_al)
  SOGI/4(q_be) -> Sequence Comps/4(qv_be)
  Sequence Comps/1(v_al_pos) -> v_al_pos/1
  Sequence Comps/3(v_al_neg) -> v_al_neg/1
  w_est/1 -> SOGI/4(w_est)
  vc/1 -> Data Type Conversion2/1
  vb/1 -> Data Type Conversion1/1
  va/1 -> Data Type Conversion/1
  Data Type Conversion/1 -> SOGI/1(va)
  Data Type Conversion1/1 -> SOGI/2(vb)
  Data Type Conversion2/1 -> SOGI/3(vc)

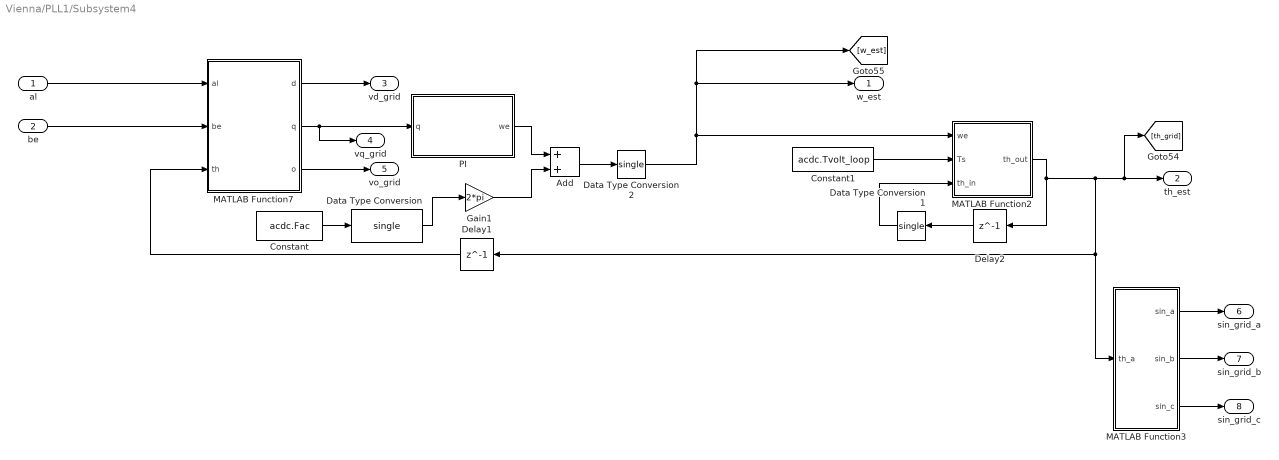
== system Vienna/PLL1/Subsystem4 ==
  al : Inport
  be : Inport  Port=2
  Add : Sum  AccumDataTypeStr=single
  Constant : Constant  Value=acdc.Fac
  Constant1 : Constant  Value=acdc.Tvolt_loop  OutDataTypeStr=single
  Data Type Conversion : DataTypeConversion  OutDataTypeStr=single  SaturateOnIntegerOverflow=off  RndMeth=Floor
  Data Type Conversion1 : DataTypeConversion  OutDataTypeStr=single  SaturateOnIntegerOverflow=off  RndMeth=Floor
  Data Type Conversion2 : DataTypeConversion  OutDataTypeStr=single  SaturateOnIntegerOverflow=off  RndMeth=Floor
  Delay1 : Delay  DelayLength=1
  Delay2 : Delay  DelayLength=1
  Gain1 : Gain  Gain=2*pi
  MATLAB Function2 : MATLAB Function  TreatAsAtomicUnit=on
  MATLAB Function3 : MATLAB Function  TreatAsAtomicUnit=on
  MATLAB Function7 : MATLAB Function  TreatAsAtomicUnit=on
  PI : Subsystem
  w_est : Outport
  th_est : Outport  Port=2
  vd_grid : Outport  Port=3
  vq_grid : Outport  Port=4
  vo_grid : Outport  Port=5
  sin_grid_a : Outport  Port=6
  sin_grid_b : Outport  Port=7
  sin_grid_c : Outport  Port=8
  wires:
  MATLAB Function2/1(th_out) -> th_est/1, [th_grid], MATLAB Function3/1(th_a), Delay1/1, Delay2/1
  Gain1/1 -> Add/2
  Constant/1 -> Data Type Conversion/1
  MATLAB Function3/1(sin_a) -> sin_grid_a/1
  MATLAB Function7/3(o) -> vo_grid/1
  Add/1 -> Data Type Conversion2/1
  MATLAB Function7/2(q) -> vq_grid/1, PI/1(q)
  Delay1/1 -> MATLAB Function7/3(th)
  Constant1/1 -> MATLAB Function2/2(Ts)
  MATLAB Function3/3(sin_c) -> sin_grid_c/1
  al/1 -> MATLAB Function7/1(al)
  Delay2/1 -> Data Type Conversion1/1
  MATLAB Function3/2(sin_b) -> sin_grid_b/1
  PI/1(we) -> Add/1
  MATLAB Function7/1(d) -> vd_grid/1
  be/1 -> MATLAB Function7/2(be)
  Data Type Conversion/1 -> Gain1/1
  Data Type Conversion1/1 -> MATLAB Function2/3(th_in)
  Data Type Conversion2/1 -> w_est/1, [w_est], MATLAB Function2/1(we)

== system Vienna/Subsystem/Variant Subsystem ==
  va_duty : Inport
  vb_duty : Inport  Port=2
  vc_duty : Inport  Port=3
  car : Inport  Port=4
  Subsystem : Subsystem  VariantControl=PWM_strategy == 1
  Subsystem1 : Subsystem  VariantControl=PWM_strategy == 0
  PWM1 : Outport
  PWM2 : Outport  Port=2
  PWM3 : Outport  Port=3
  PWM4 : Outport  Port=4
  PWM5 : Outport  Port=5
  PWM6 : Outport  Port=6

== system Vienna/Subsystem1/Subsystem ==
  s : Inport
  s1 : Inport  Port=2
  s2 : Inport  Port=3
  Controlled Voltage Source1 : spsControlledVoltageSourceLib/Controlled Voltage Source  Initialize=on  Source_Type=AC  Amplitude=0  Phase=0  Frequency=0  Measurements=None
  Controlled Voltage Source2 : spsControlledVoltageSourceLib/Controlled Voltage Source  Initialize=on  Source_Type=AC  Amplitude=0  Phase=0  Frequency=0  Measurements=None
  Controlled Voltage Source3 : spsControlledVoltageSourceLib/Controlled Voltage Source  Initialize=on  Source_Type=AC  Amplitude=0  Phase=0  Frequency=0  Measurements=None
  A : PMIOPort  Side=Right
  B : PMIOPort  Port=2  Side=Right
  C : PMIOPort  Port=3  Side=Right
  N : PMIOPort  Port=4  Side=Right
  wires:
  s/1 -> Controlled Voltage Source3/1
  s1/1 -> Controlled Voltage Source1/1
  s2/1 -> Controlled Voltage Source2/1
  connections:
  Controlled Voltage Source3/LConn1 -- N/RConn1 -- Controlled Voltage Source2/LConn1 -- Controlled Voltage Source1/LConn1
  Controlled Voltage Source2/RConn1 -- C/RConn1
  Controlled Voltage Source3/RConn1 -- A/RConn1
  Controlled Voltage Source1/RConn1 -- B/RConn1

== system Vienna/Subsystem1/Subsystem1 ==
  Add : Sum  Inputs=+++
  Add1 : Sum  Inputs=+++
  Add2 : Sum  Inputs=+++
  Sine Wave : Sin  Amplitude=acdc.va_pk  Frequency=acdc.Wac  Phase=acdc.va_ph_rad  SampleTime=0
  Sine Wave1 : Sin  Amplitude=acdc.va_pk_3rd  Frequency=acdc.Wac*3  Phase=acdc.va_ph_rad  SampleTime=0
  Sine Wave2 : Sin  Amplitude=acdc.va_pk_5th  Frequency=acdc.Wac*5  Phase=acdc.va_ph_rad  SampleTime=0
  Sine Wave3 : Sin  Amplitude=acdc.vb_pk  Frequency=acdc.Wac  Phase=acdc.vb_ph_rad  SampleTime=0
  Sine Wave4 : Sin  Amplitude=acdc.vb_pk_3rd  Frequency=acdc.Wac*3  Phase=acdc.vb_ph_rad*3  SampleTime=0
  Sine Wave5 : Sin  Amplitude=acdc.vb_pk_5th  Frequency=acdc.Wac*5  Phase=acdc.vb_ph_rad*5  SampleTime=0
  Sine Wave6 : Sin  Amplitude=acdc.vc_pk  Frequency=acdc.Wac  Phase=acdc.vc_ph_rad  SampleTime=0
  Sine Wave7 : Sin  Amplitude=acdc.vc_pk_3rd  Frequency=acdc.Wac*3  Phase=acdc.vc_ph_rad*3  SampleTime=0
  Sine Wave8 : Sin  Amplitude=acdc.vc_pk_5th  Frequency=acdc.Wac*5  Phase=acdc.vc_ph_rad*5  SampleTime=0
  s : Outport
  s1 : Outport  Port=2
  s2 : Outport  Port=3
  wires:
  Add/1 -> s/1
  Sine Wave1/1 -> Add/2
  Sine Wave2/1 -> Add/3
  Sine Wave/1 -> Add/1
  Sine Wave3/1 -> Add1/1
  Sine Wave5/1 -> Add1/3
  Sine Wave4/1 -> Add1/2
  Sine Wave6/1 -> Add2/1
  Sine Wave8/1 -> Add2/3
  Sine Wave7/1 -> Add2/2
  Add1/1 -> s1/1
  Add2/1 -> s2/1

== system Vienna/Variant Subsystem/S FUNCTION CONTROL ==
  duty_a : Inport
  duty_b : Inport  Port=2
  duty_c : Inport  Port=3
  duty_a_sf : Inport  Port=4
  duty_b_sf : Inport  Port=5
  duty_c_sf : Inport  Port=6
  Terminator : Terminator
  Terminator1 : Terminator
  Terminator2 : Terminator
  dutyA : Outport
  dutyB : Outport  Port=2
  dutyC : Outport  Port=3
  wires:
  duty_a_sf/1 -> dutyA/1
  duty_b_sf/1 -> dutyB/1
  duty_c_sf/1 -> dutyC/1
  duty_a/1 -> Terminator/1
  duty_b/1 -> Terminator1/1
  duty_c/1 -> Terminator2/1

== system Vienna/Variant Subsystem/SIMULINK BLOCK CONTROL ==
  duty_a : Inport
  duty_b : Inport  Port=2
  duty_c : Inport  Port=3
  duty_a_sf : Inport  Port=4
  duty_b_sf : Inport  Port=5
  duty_c_sf : Inport  Port=6
  Terminator : Terminator
  Terminator1 : Terminator
  Terminator2 : Terminator
  dutyA : Outport
  dutyB : Outport  Port=2
  dutyC : Outport  Port=3
  wires:
  duty_a/1 -> dutyA/1
  duty_b/1 -> dutyB/1
  duty_c/1 -> dutyC/1
  duty_a_sf/1 -> Terminator/1
  duty_b_sf/1 -> Terminator1/1
  duty_c_sf/1 -> Terminator2/1

== system Vienna/Vbus_Controller/PI ==
  q : Inport
  Add : Sum
  Discrete-Time Integrator : DiscreteIntegrator  SampleTime=-1  LimitOutput=on  UpperSaturationLimit=acdc.vdc_con_max  LowerSaturationLimit=acdc.vdc_con_min  ICPrevOutput=DiscIntNeverNeededParam  ICPrevScaledInput=DiscIntNeverNeededParam
  Gain : Gain  Gain=acdc.vdc_ki
  Gain1 : Gain  Gain=acdc.vdc_kp
  Saturation : Saturate  UpperLimit=acdc.vdc_con_max  LowerLimit=acdc.vdc_con_min
  Out1 : Outport
  wires:
  Gain1/1 -> Add/1
  Saturation/1 -> Out1/1
  Add/1 -> Saturation/1
  q/1 -> Gain1/1, Gain/1
  Gain/1 -> Discrete-Time Integrator/1
  Discrete-Time Integrator/1 -> Add/2

== system Vienna/Current Ref Generation/Variant Subsystem/current control ==
  grid_a_sin : Inport
  grid_b_sin : Inport  Port=2
  grid_c_sin : Inport  Port=3
  vdc_con_out : Inport  Port=4
  Product : Product
  Product1 : Product
  Product2 : Product
  ia_ref : Outport
  ib_ref : Outport  Port=2
  ic_ref : Outport  Port=3
  wires:
  grid_a_sin/1 -> Product/1
  vdc_con_out/1 -> Product2/2, Product1/2, Product/2
  Product/1 -> ia_ref/1
  grid_b_sin/1 -> Product1/1
  Product1/1 -> ib_ref/1
  grid_c_sin/1 -> Product2/1
  Product2/1 -> ic_ref/1

== system Vienna/Current Ref Generation/Variant Subsystem/power control ==
  va : Inport
  vb : Inport  Port=2
  vc : Inport  Port=3
  vdc_con_out : Inport  Port=4
  MATLAB Function4 : MATLAB Function  TreatAsAtomicUnit=on
  ia_ref : Outport
  ib_ref : Outport  Port=2
  ic_ref : Outport  Port=3
  wires:
  va/1 -> [va]
  vdc_con_out/1 -> [Pin]
  vb/1 -> [vb]
  vc/1 -> [vc]
  [va] -> MATLAB Function4/1(va)
  [vb] -> MATLAB Function4/2(vb)
  [vc] -> MATLAB Function4/3(vc)
  [Pin] -> MATLAB Function4/4(Pin)
  MATLAB Function4/1(ia) -> ia_ref/1
  MATLAB Function4/2(ib) -> ib_ref/1
  MATLAB Function4/3(ic) -> ic_ref/1

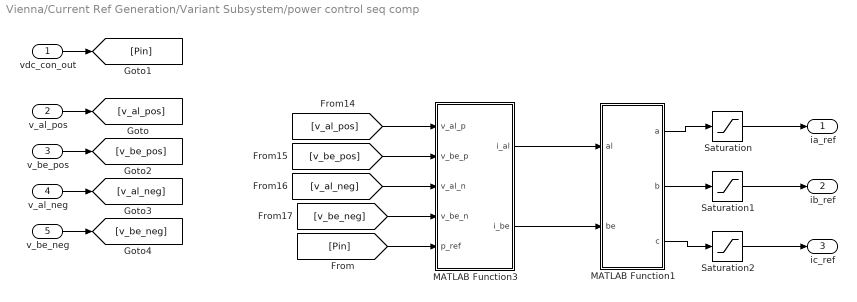
== system Vienna/Current Ref Generation/Variant Subsystem/power control seq comp ==
  vdc_con_out : Inport
  v_al_pos : Inport  Port=2
  v_be_pos : Inport  Port=3
  v_al_neg : Inport  Port=4
  v_be_neg : Inport  Port=5
  MATLAB Function1 : MATLAB Function  TreatAsAtomicUnit=on
  MATLAB Function3 : MATLAB Function  TreatAsAtomicUnit=on
  Saturation : Saturate  UpperLimit=acdc.Igrid_ph_pk*1.5  LowerLimit=-acdc.Igrid_ph_pk*1.5  OutDataTypeStr=single
  Saturation1 : Saturate  UpperLimit=acdc.Igrid_ph_pk*1.5  LowerLimit=-acdc.Igrid_ph_pk*1.5  OutDataTypeStr=single
  Saturation2 : Saturate  UpperLimit=acdc.Igrid_ph_pk*1.5  LowerLimit=-acdc.Igrid_ph_pk*1.5  OutDataTypeStr=single
  ia_ref : Outport
  ib_ref : Outport  Port=2
  ic_ref : Outport  Port=3
  wires:
  vdc_con_out/1 -> [Pin]
  MATLAB Function3/2(i_be) -> MATLAB Function1/2(be)
  [v_be_pos] -> MATLAB Function3/2(v_be_p)
  MATLAB Function1/1(a) -> Saturation/1
  [v_al_neg] -> MATLAB Function3/3(v_al_n)
  [v_al_pos] -> MATLAB Function3/1(v_al_p)
  MATLAB Function3/1(i_al) -> MATLAB Function1/1(al)
  MATLAB Function1/2(b) -> Saturation1/1
  Saturation1/1 -> ib_ref/1
  [v_be_neg] -> MATLAB Function3/4(v_be_n)
  Saturation/1 -> ia_ref/1
  [Pin] -> MATLAB Function3/5(p_ref)
  Saturation2/1 -> ic_ref/1
  MATLAB Function1/3(c) -> Saturation2/1
  v_al_pos/1 -> [v_al_pos]
  v_be_pos/1 -> [v_be_pos]
  v_al_neg/1 -> [v_al_neg]
  v_be_neg/1 -> [v_be_neg]

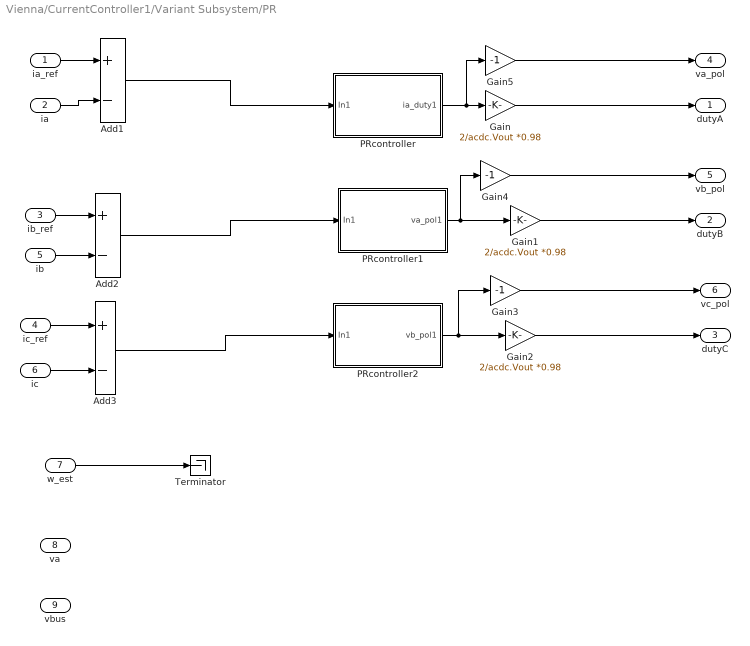
== system Vienna/CurrentController1/Variant Subsystem/PR ==
  ia_ref : Inport
  ia : Inport  Port=2
  ib_ref : Inport  Port=3
  ic_ref : Inport  Port=4
  ib : Inport  Port=5
  ic : Inport  Port=6
  w_est : Inport  Port=7
  va : Inport  Port=8
  vbus : Inport  Port=9
  Add1 : Sum  Inputs=+-
  Add2 : Sum  Inputs=+-
  Add3 : Sum  Inputs=+-
  Gain : Gain  Gain=2/acdc.Vout *0.98
  Gain1 : Gain  Gain=2/acdc.Vout *0.98
  Gain2 : Gain  Gain=2/acdc.Vout *0.98
  Gain3 : Gain  Gain=-1
  Gain4 : Gain  Gain=-1
  Gain5 : Gain  Gain=-1
  PRcontroller : Subsystem
  PRcontroller1 : Subsystem
  PRcontroller2 : Subsystem
  Terminator : Terminator
  dutyA : Outport
  dutyB : Outport  Port=2
  dutyC : Outport  Port=3
  va_pol : Outport  Port=4
  vb_pol : Outport  Port=5
  vc_pol : Outport  Port=6
  wires:
  PRcontroller2/1(vb_pol1) -> Gain3/1, Gain2/1
  Add3/1 -> PRcontroller2/1(In1)
  PRcontroller/1(ia_duty1) -> Gain5/1, Gain/1
  PRcontroller1/1(va_pol1) -> Gain4/1, Gain1/1
  Add1/1 -> PRcontroller/1(In1)
  Add2/1 -> PRcontroller1/1(In1)
  ia/1 -> Add1/2
  ia_ref/1 -> Add1/1
  ic_ref/1 -> Add3/1
  ib_ref/1 -> Add2/1
  ib/1 -> Add2/2
  ic/1 -> Add3/2
  w_est/1 -> Terminator/1
  Gain/1 -> dutyA/1
  Gain1/1 -> dutyB/1
  Gain2/1 -> dutyC/1
  Gain5/1 -> va_pol/1
  Gain4/1 -> vb_pol/1
  Gain3/1 -> vc_pol/1

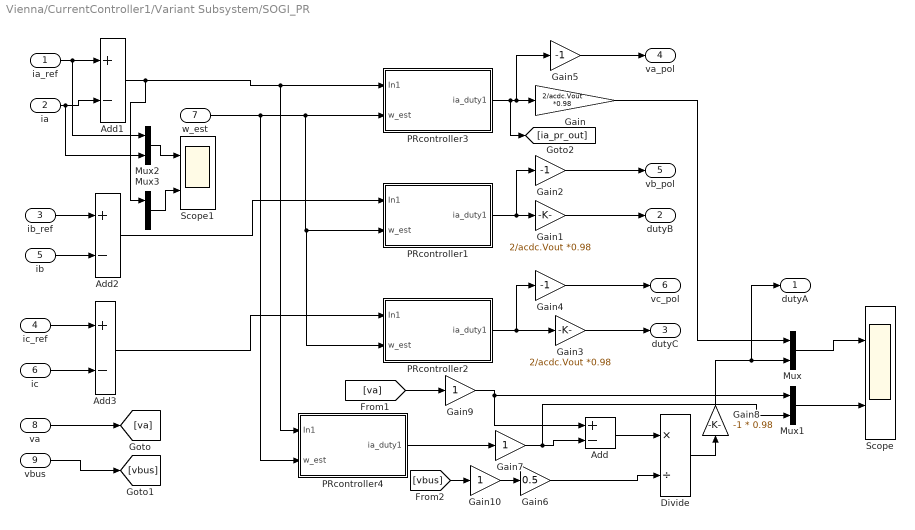
== system Vienna/CurrentController1/Variant Subsystem/SOGI_PR ==
  ia_ref : Inport
  ia : Inport  Port=2
  ib_ref : Inport  Port=3
  ic_ref : Inport  Port=4
  ib : Inport  Port=5
  ic : Inport  Port=6
  w_est : Inport  Port=7
  va : Inport  Port=8
  vbus : Inport  Port=9
  Add{,1..3} (4 alike) : Sum  Inputs=+-
  Divide : Product  Inputs=*/
  Gain : Gain  Gain=2/acdc.Vout *0.98
  Gain1 : Gain  Gain=2/acdc.Vout *0.98
  Gain10 : Gain
  Gain2 : Gain  Gain=-1
  Gain3 : Gain  Gain=2/acdc.Vout *0.98
  Gain4 : Gain  Gain=-1
  Gain5 : Gain  Gain=-1
  Gain6 : Gain  Gain=0.5
  Gain7 : Gain
  Gain8 : Gain  Gain=-1 * 0.98
  Gain9 : Gain
  Mux{,1..3} (4 alike) : Mux  Inputs=2
  PRcontroller1 : Subsystem
  PRcontroller2 : Subsystem
  PRcontroller3 : Subsystem
  PRcontroller4 : Subsystem
  Scope : Scope  NumInputPorts=2
  Scope1 : Scope  NumInputPorts=2
  dutyA : Outport
  dutyB : Outport  Port=2
  dutyC : Outport  Port=3
  va_pol : Outport  Port=4
  vb_pol : Outport  Port=5
  vc_pol : Outport  Port=6
  wires:
  PRcontroller2/1(ia_duty1) -> Gain4/1, Gain3/1
  PRcontroller3/1(ia_duty1) -> Gain/1, Gain5/1, [ia_pr_out]
  Gain3/1 -> dutyC/1
  Gain2/1 -> vb_pol/1
  PRcontroller1/1(ia_duty1) -> Gain2/1, Gain1/1
  Gain/1 -> Mux/1
  Gain5/1 -> va_pol/1
  Gain1/1 -> dutyB/1
  Gain4/1 -> vc_pol/1
  ia_ref/1 -> Mux2/1, Add1/1
  ia/1 -> Mux2/2, Add1/2
  ic_ref/1 -> Add3/1
  ic/1 -> Add3/2
  ib_ref/1 -> Add2/1
  ib/1 -> Add2/2
  Add1/1 -> Mux3/1, PRcontroller3/1(In1), PRcontroller4/1(In1)
  Add2/1 -> PRcontroller1/1(In1)
  Add3/1 -> PRcontroller2/1(In1)
  w_est/1 -> PRcontroller4/2(w_est), PRcontroller2/2(w_est), PRcontroller1/2(w_est), PRcontroller3/2(w_est)
  va/1 -> [va]
  vbus/1 -> [vbus]
  [va] -> Gain9/1
  PRcontroller4/1(ia_duty1) -> Gain7/1
  Add/1 -> Divide/1
  [vbus] -> Gain10/1
  Mux/1 -> Scope/1
  Mux1/1 -> Scope/2
  Divide/1 -> Gain8/1
  Gain6/1 -> Divide/2
  Gain7/1 -> Mux1/2, Add/2
  Gain8/1 -> dutyA/1, Mux/2
  Mux3/1 -> Scope1/2
  Mux2/1 -> Scope1/1
  Gain9/1 -> Add/1, Mux1/1
  Gain10/1 -> Gain6/1

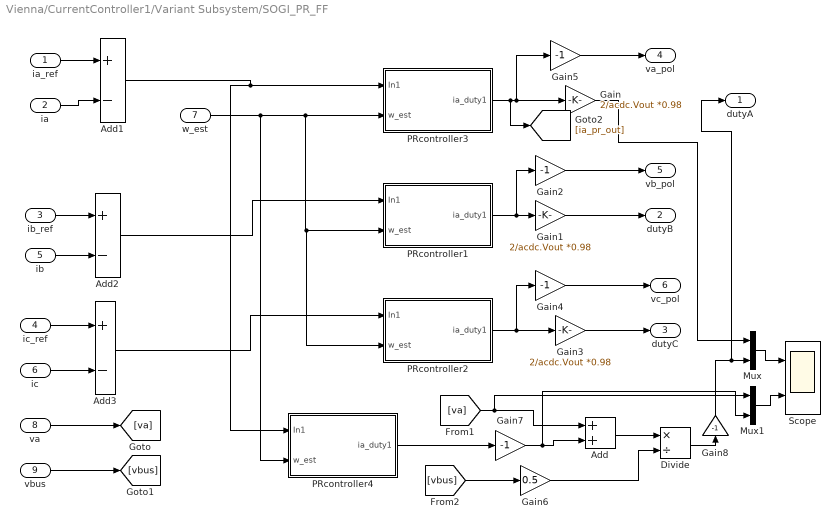
== system Vienna/CurrentController1/Variant Subsystem/SOGI_PR_FF ==
  ia_ref : Inport
  ia : Inport  Port=2
  ib_ref : Inport  Port=3
  ic_ref : Inport  Port=4
  ib : Inport  Port=5
  ic : Inport  Port=6
  w_est : Inport  Port=7
  va : Inport  Port=8
  vbus : Inport  Port=9
  Add : Sum
  Add1 : Sum  Inputs=+-
  Add2 : Sum  Inputs=+-
  Add3 : Sum  Inputs=+-
  Divide : Product  Inputs=*/
  Gain : Gain  Gain=2/acdc.Vout *0.98
  Gain1 : Gain  Gain=2/acdc.Vout *0.98
  Gain{2,4..5,7..8} (5 alike) : Gain  Gain=-1
  Gain3 : Gain  Gain=2/acdc.Vout *0.98
  Gain6 : Gain  Gain=0.5
  Mux : Mux  Inputs=2
  Mux1 : Mux  Inputs=2
  PRcontroller1 : Subsystem
  PRcontroller2 : Subsystem
  PRcontroller3 : Subsystem
  PRcontroller4 : Subsystem
  Scope : Scope  NumInputPorts=2
  dutyA : Outport
  dutyB : Outport  Port=2
  dutyC : Outport  Port=3
  va_pol : Outport  Port=4
  vb_pol : Outport  Port=5
  vc_pol : Outport  Port=6
  wires:
  PRcontroller2/1(ia_duty1) -> Gain4/1, Gain3/1
  PRcontroller3/1(ia_duty1) -> Gain/1, Gain5/1, [ia_pr_out]
  Gain3/1 -> dutyC/1
  Gain2/1 -> vb_pol/1
  PRcontroller1/1(ia_duty1) -> Gain2/1, Gain1/1
  Gain/1 -> Mux/1
  Gain5/1 -> va_pol/1
  Gain1/1 -> dutyB/1
  Gain4/1 -> vc_pol/1
  ia_ref/1 -> Add1/1
  ia/1 -> Add1/2
  ic_ref/1 -> Add3/1
  ic/1 -> Add3/2
  ib_ref/1 -> Add2/1
  ib/1 -> Add2/2
  Add1/1 -> PRcontroller3/1(In1), PRcontroller4/1(In1)
  Add2/1 -> PRcontroller1/1(In1)
  Add3/1 -> PRcontroller2/1(In1)
  w_est/1 -> PRcontroller4/2(w_est), PRcontroller2/2(w_est), PRcontroller1/2(w_est), PRcontroller3/2(w_est)
  va/1 -> [va]
  vbus/1 -> [vbus]
  [va] -> Mux1/1, Add/1
  PRcontroller4/1(ia_duty1) -> Gain7/1
  Add/1 -> Divide/1
  [vbus] -> Gain6/1
  Mux/1 -> Scope/1
  Mux1/1 -> Scope/2
  Divide/1 -> Gain8/1
  Gain6/1 -> Divide/2
  Gain7/1 -> Mux1/2, Add/2
  Gain8/1 -> dutyA/1, Mux/2

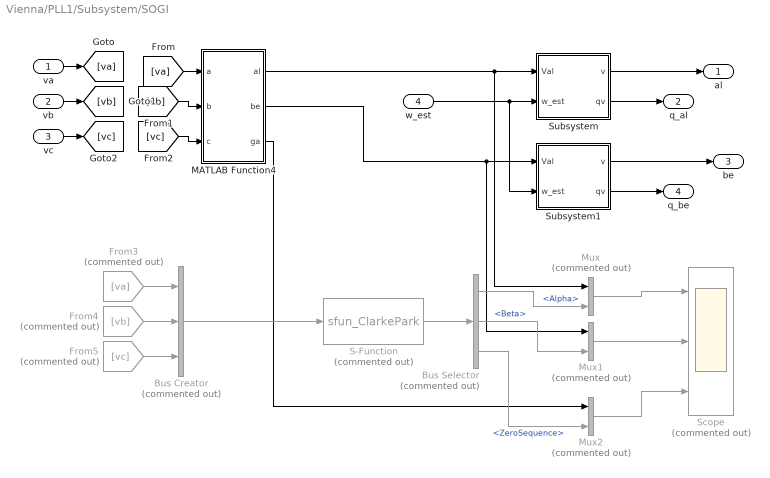
== system Vienna/PLL1/Subsystem/SOGI ==
  va : Inport
  vb : Inport  Port=2
  vc : Inport  Port=3
  w_est : Inport  Port=4
  Bus Creator : BusCreator  Commented=on  Inputs=3
  Bus Selector : BusSelector  Commented=on  OutputSignals=Alpha,Beta,ZeroSequence
  From3 : From  Commented=on  GotoTag=va
  From4 : From  Commented=on  GotoTag=vb
  From5 : From  Commented=on  GotoTag=vc
  MATLAB Function4 : MATLAB Function  TreatAsAtomicUnit=on
  Mux : Mux  Commented=on  Inputs=2
  Mux1 : Mux  Commented=on  Inputs=2
  Mux2 : Mux  Commented=on  Inputs=2
  S-Function : S-Function  Commented=on  FunctionName=sfun_ClarkePark  SFunctionDeploymentMode=off  EnableBusSupport=off
  Scope : Scope  Commented=on  NumInputPorts=3
  Subsystem : Subsystem
  Subsystem1 : Subsystem
  al : Outport
  q_al : Outport  Port=2
  be : Outport  Port=3
  q_be : Outport  Port=4
  wires:
  MATLAB Function4/1(al) -> Mux/1, Subsystem/1(Val)
  Subsystem/1(v) -> al/1
  Subsystem/2(qv) -> q_al/1
  Subsystem1/2(qv) -> q_be/1
  MATLAB Function4/2(be) -> Mux1/1, Subsystem1/1(Val)
  w_est/1 -> Subsystem1/2(w_est), Subsystem/2(w_est)
  Subsystem1/1(v) -> be/1
  MATLAB Function4/3(ga) -> Mux2/1
  Bus Creator/1 -> S-Function/1
  va/1 -> [va]
  vb/1 -> [vb]
  vc/1 -> [vc]
  [va] -> MATLAB Function4/1(a)
  [vb] -> MATLAB Function4/2(b)
  [vc] -> MATLAB Function4/3(c)
  From3/1 -> Bus Creator/1
  From4/1 -> Bus Creator/2
  From5/1 -> Bus Creator/3
  S-Function/1 -> Bus Selector/1
  Bus Selector/1 -> Mux/2  "<Alpha>"
  Bus Selector/2 -> Mux1/2  "<Beta>"
  Mux/1 -> Scope/1
  Mux1/1 -> Scope/2
  Bus Selector/3 -> Mux2/2  "<ZeroSequence>"
  Mux2/1 -> Scope/3

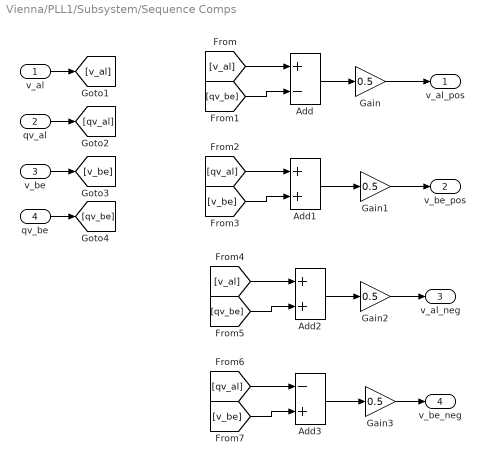
== system Vienna/PLL1/Subsystem/Sequence Comps ==
  v_al : Inport
  qv_al : Inport  Port=2
  v_be : Inport  Port=3
  qv_be : Inport  Port=4
  Add : Sum  Inputs=+-
  Add1 : Sum
  Add2 : Sum
  Add3 : Sum  Inputs=-+
  Gain{,1..3} (4 alike) : Gain  Gain=0.5
  v_al_pos : Outport
  v_be_pos : Outport  Port=2
  v_al_neg : Outport  Port=3
  v_be_neg : Outport  Port=4
  wires:
  qv_al/1 -> [qv_al]
  v_al/1 -> [v_al]
  v_be/1 -> [v_be]
  qv_be/1 -> [qv_be]
  Add1/1 -> Gain1/1
  Add/1 -> Gain/1
  [v_al] -> Add/1
  [qv_be] -> Add/2
  [qv_al] -> Add1/1
  [v_be] -> Add1/2
  Gain/1 -> v_al_pos/1
  Gain1/1 -> v_be_pos/1
  Add2/1 -> Gain2/1
  Add3/1 -> Gain3/1
  [v_be] -> Add3/2
  [qv_be] -> Add2/2
  [qv_al] -> Add3/1
  [v_al] -> Add2/1
  Gain3/1 -> v_be_neg/1
  Gain2/1 -> v_al_neg/1

== system Vienna/PLL1/Subsystem4/PI ==
  q : Inport
  Add : Sum
  Discrete-Time Integrator : DiscreteIntegrator  SampleTime=-1  LimitOutput=on  UpperSaturationLimit=2*pi*acdc.Fac*1.2  LowerSaturationLimit=-2*pi*acdc.Fac*1.2  ICPrevOutput=DiscIntNeverNeededParam  ICPrevScaledInput=DiscIntNeverNeededParam
  Gain : Gain  Gain=50
  Gain1 : Gain  Gain=3
  Saturation : Saturate  UpperLimit=2*pi*acdc.Fac*1.2  LowerLimit=-2*pi*acdc.Fac*1.2
  Scope4 : Scope  NumInputPorts=3
  we : Outport
  wires:
  Gain1/1 -> Scope4/1, Add/1
  Saturation/1 -> we/1
  Add/1 -> Scope4/3, Saturation/1
  q/1 -> Gain1/1, Gain/1
  Gain/1 -> Discrete-Time Integrator/1
  Discrete-Time Integrator/1 -> Scope4/2, Add/2
